simulink model "CopterSim3DEnvironment123"  (R2022a)
settings: Solver=ode4  StartTime=0.0  StopTime=2000  FixedStep=0.001  RelTol=1e-3
PreLoadFcn:
  | filepath  = fileparts(get_param(bdroot, 'FileName'));
  | cd(filepath);
InitFcn:
  | if exist('Init_control.m','file')
  |      Init_control;
  | end
undefined symbols (not defined in the file): d_i, Earth, earthRadius, h_i, KiPitchAttitude, KiPitchRate, KiRollAttitude, KiRollRate, KiYawRate, KpPitchAttitude, KpPitchRate, KpRollAttitude, KpRollRate, KpYawRate, ModelInit_RPM, ModelParam_envAltitude, ModelParam_GlobalNoiseGainSwitch, ModelParam_GPSEphFinal, ModelParam_GPSEpvFinal, ModelParam_GPSEpvInitial, ModelParam_GPSEpvTimeConstant, ModelParam_GPSFix3DFix, ModelParam_GPSSatsVisible, ModelParam_motorCr, ModelParam_motorJm, ModelParam_motorMinThr, ModelParam_motorT, ModelParam_motorWb, ModelParam_noiseBaroCoupleWithSpeed, ModelParam_noiseGPSSampTime, ModelParam_noiseLowPassFilterCoeAccel, ModelParam_noiseLowPassFilterCoeGyro, ModelParam_noisePowerIMU, ModelParam_noisePowerOffGainAccel, ModelParam_noisePowerOffGainAccelZ, ModelParam_noisePowerOffGainGyro, ModelParam_noisePowerOffGainGyroZ, ModelParam_noisePowerOffGainMag, ModelParam_noisePowerOffGainMagZ, ModelParam_noisePowerOnGainAccel, ModelParam_noisePowerOnGainAccelZ, ModelParam_noisePowerOnGainGyro, ModelParam_noisePowerOnGainGyroZ, ModelParam_noisePowerOnGainMag, ModelParam_noisePowerOnGainMagZ, ModelParam_noiseSampleTimeAccel, ModelParam_noiseSampleTimeGyro, ModelParam_noiseSampleTimeMag, ModelParam_noiseUpperGPS, ModelParam_noiseUpperWindBodyRatio, ModelParam_noiseWindSampTime, ModelParam_rotorCm, ModelParam_rotorCt, ModelParam_timeSamp, ModelParam_timeSampBaro, ModelParam_uavCCm, ModelParam_uavCd, ModelParam_uavDearo, ModelParam_uavMass, ModelParam_uavR ... (+6)
libraries: simulink x12, slpidlib x5, aerolibfltsims x4, aerolibtransform2 x3, sharedtransform x3, aerolibasang x3, aerolibatmos2 x2, sharedutil x2, aerolibutil x2, etargetslib x2, shared6dof x1, aerolibconvert2 x1
(part 2 of 3)

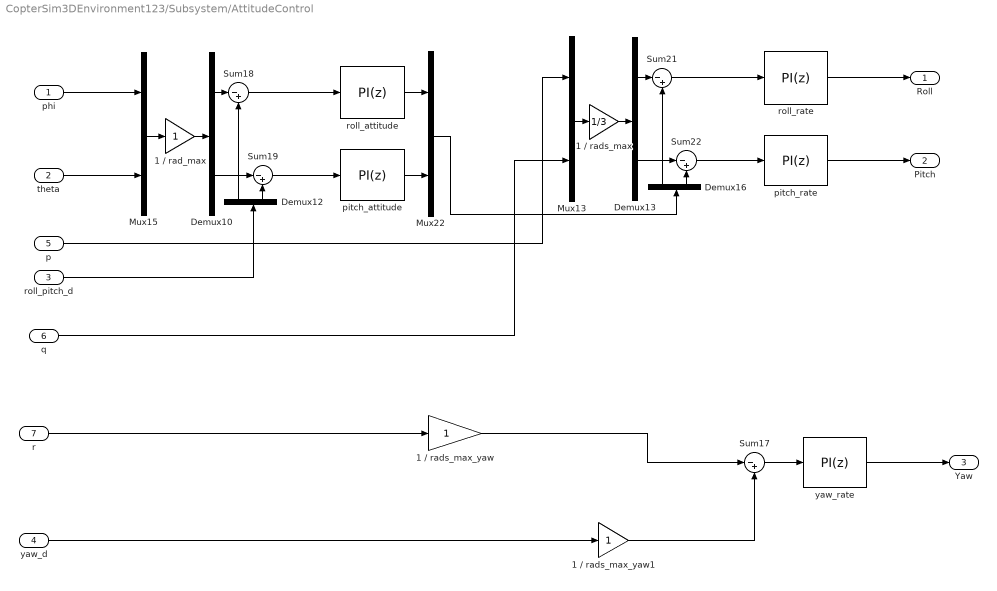
== system CopterSim3DEnvironment123/Subsystem/AttitudeControl ==
  phi : Inport
  theta : Inport  Port=2
  roll_pitch_d : Inport  Port=3
  yaw_d : Inport  Port=4
  p : Inport  Port=5
  q : Inport  Port=6
  r : Inport  Port=7
  1 / rad_max : Gain
  1 / rads_max : Gain  Gain=1/3
  1 / rads_max_yaw : Gain
  1 / rads_max_yaw1 : Gain
  Demux{10,12..13,16} (4 alike) : Demux  Outputs=2
  Mux13 : Mux  Inputs=2
  Mux15 : Mux  Inputs=2
  Mux22 : Mux  Inputs=2
  Sum{17..19,21..22} (5 alike) : Sum  Inputs=|-+
  pitch_attitude : slpidlib/PID Controller  Controller=PI  Form=Parallel  TimeDomain=Discrete-time  UseExternalTs=off  SampleTime=-1  IntegratorMethod=Forward Euler  FilterMethod=Forward Euler  ControllerParametersSource=internal  P=KpPitchAttitude  I=KiPitchAttitude  UseKiTs=off  D=0.01  N=100  UseFilter=on  TunerSelectOption=Transfer Function Based (PID Tuner App)  InitialConditionSource=internal  InitialConditionForIntegrator=0  InitialConditionForFilter=0  DifferentiatorICPrevScaledInput=0  ExternalReset=none  TrackingMode=off  Kt=1  LimitOutput=on  SatLimitsSource=internal  UpperSaturationLimit=1  LowerSaturationLimit=-1  LinearizeAsGain=on  AntiWindupMode=back-calculation  Kb=1  POutMin=[]  POutMax=[]  IOutMin=[]  IOutMax=[]  DOutMin=[]  DOutMax=[]  NOutMin=[]  NOutMax=[]  SumOutMin=[]  SumOutMax=[]  SaturationOutMin=[]  SaturationOutMax=[]  PParamMin=[]  PParamMax=[]  IParamMin=[]  IParamMax=[]  DParamMin=[]  DParamMax=[]  NParamMin=[]  NParamMax=[]  KbParamMin=[]  KbParamMax=[]  KtParamMin=[]  KtParamMax=[]  KbOutMin=[]  KbOutMax=[]  KtOutMin=[]  KtOutMax=[]  IntegratorOutMin=[]  IntegratorOutMax=[]  FilterOutMin=[]  FilterOutMax=[]  SumI1OutMin=[]  SumI1OutMax=[]  SumI2OutMin=[]  SumI2OutMax=[]  SumI3OutMin=[]  SumI3OutMax=[]  SumI4OutMin=[]  SumI4OutMax=[]  SumDOutMin=[]  SumDOutMax=[]  DifferentiatorOutMin=[]  DifferentiatorOutMax=[]  FilterDiffOutCoefMin=[]  FilterDiffOutCoefMax=[]  ReciprocalOutMin=[]  ReciprocalOutMax=[]  SumDenOutMin=[]  SumDenOutMax=[]  SumNumOutMin=[]  SumNumOutMax=[]  DivideOutMin=[]  DivideOutMax=[]  UdiffTsProdOutMin=[]  UdiffTsProdOutMax=[]  NTsProdOutMin=[]  NTsProdOutMax=[]  UintegralTsProdOutMin=[]  UintegralTsProdOutMax=[]  UngainTsProdOutMin=[]  UngainTsProdOutMax=[]  IntegratorContinuousStateAttributes=''  IntegratorStateMustResolveToSignalObject=off  IntegratorRTWStateStorageClass=Auto  FilterContinuousStateAttributes=''  FilterStateMustResolveToSignalObject=off  FilterRTWStateStorageClass=Auto  ParallelPVariant=InternalParameters  IdealPVariant=Disabled  IVariant=InternalParameters  DVariant=Disabled  IntegratorVariant=Discrete  SatVariant=Enabled  AWVariant=BackCalculation  PCopyVariant=Disabled  TRVariant=Disabled  FdbkBlocksVariant=Forward  IdealPFdbkVariant=Disabled  SatFdbkVariant=Disabled  DerivativeFilterVariant=Disabled  NVariant=Disabled  NCopyVariant=Disabled_SignalSpec  FilterICVariant=Disabled  IntegratorICVariant=InternalICs  ExternalResetVariant=Disabled  TRSumVariant=Passthrough  SumFdbkVariant=Disabled  SumVariant=Sum_PI  TsampFilterVariant=InternalTs  TsampNgainVariant=Passthrough  TsampIntegralVariant=Passthrough  ExternalSaturationOutDataTypeStr=Inherit: Same as second input  aMode=0
  pitch_rate : slpidlib/PID Controller  Controller=PI  Form=Parallel  TimeDomain=Discrete-time  UseExternalTs=off  SampleTime=-1  IntegratorMethod=Forward Euler  FilterMethod=Forward Euler  ControllerParametersSource=internal  P=KpPitchRate  I=KiPitchRate  UseKiTs=off  D=0.0024  N=100  UseFilter=on  TunerSelectOption=Transfer Function Based (PID Tuner App)  InitialConditionSource=internal  InitialConditionForIntegrator=0  InitialConditionForFilter=0  DifferentiatorICPrevScaledInput=0  ExternalReset=none  TrackingMode=off  Kt=1  LimitOutput=on  SatLimitsSource=internal  UpperSaturationLimit=1  LowerSaturationLimit=-1  LinearizeAsGain=on  AntiWindupMode=back-calculation  Kb=1  POutMin=[]  POutMax=[]  IOutMin=[]  IOutMax=[]  DOutMin=[]  DOutMax=[]  NOutMin=[]  NOutMax=[]  SumOutMin=[]  SumOutMax=[]  SaturationOutMin=[]  SaturationOutMax=[]  PParamMin=[]  PParamMax=[]  IParamMin=[]  IParamMax=[]  DParamMin=[]  DParamMax=[]  NParamMin=[]  NParamMax=[]  KbParamMin=[]  KbParamMax=[]  KtParamMin=[]  KtParamMax=[]  KbOutMin=[]  KbOutMax=[]  KtOutMin=[]  KtOutMax=[]  IntegratorOutMin=[]  IntegratorOutMax=[]  FilterOutMin=[]  FilterOutMax=[]  SumI1OutMin=[]  SumI1OutMax=[]  SumI2OutMin=[]  SumI2OutMax=[]  SumI3OutMin=[]  SumI3OutMax=[]  SumI4OutMin=[]  SumI4OutMax=[]  SumDOutMin=[]  SumDOutMax=[]  DifferentiatorOutMin=[]  DifferentiatorOutMax=[]  FilterDiffOutCoefMin=[]  FilterDiffOutCoefMax=[]  ReciprocalOutMin=[]  ReciprocalOutMax=[]  SumDenOutMin=[]  SumDenOutMax=[]  SumNumOutMin=[]  SumNumOutMax=[]  DivideOutMin=[]  DivideOutMax=[]  UdiffTsProdOutMin=[]  UdiffTsProdOutMax=[]  NTsProdOutMin=[]  NTsProdOutMax=[]  UintegralTsProdOutMin=[]  UintegralTsProdOutMax=[]  UngainTsProdOutMin=[]  UngainTsProdOutMax=[]  IntegratorContinuousStateAttributes=''  IntegratorStateMustResolveToSignalObject=off  IntegratorRTWStateStorageClass=Auto  FilterContinuousStateAttributes=''  FilterStateMustResolveToSignalObject=off  FilterRTWStateStorageClass=Auto  ParallelPVariant=InternalParameters  IdealPVariant=Disabled  IVariant=InternalParameters  DVariant=Disabled  IntegratorVariant=Discrete  SatVariant=Enabled  AWVariant=BackCalculation  PCopyVariant=Disabled  TRVariant=Disabled  FdbkBlocksVariant=Forward  IdealPFdbkVariant=Disabled  SatFdbkVariant=Disabled  DerivativeFilterVariant=Disabled  NVariant=Disabled  NCopyVariant=Disabled_SignalSpec  FilterICVariant=Disabled  IntegratorICVariant=InternalICs  ExternalResetVariant=Disabled  TRSumVariant=Passthrough  SumFdbkVariant=Disabled  SumVariant=Sum_PI  TsampFilterVariant=InternalTs  TsampNgainVariant=Passthrough  TsampIntegralVariant=Passthrough  ExternalSaturationOutDataTypeStr=Inherit: Same as second input  aMode=0
  roll_attitude : slpidlib/PID Controller  Controller=PI  Form=Parallel  TimeDomain=Discrete-time  UseExternalTs=off  SampleTime=-1  IntegratorMethod=Forward Euler  FilterMethod=Forward Euler  ControllerParametersSource=internal  P=KpRollAttitude  I=KiRollAttitude  UseKiTs=off  D=0.01  N=100  UseFilter=on  TunerSelectOption=Transfer Function Based (PID Tuner App)  InitialConditionSource=internal  InitialConditionForIntegrator=0  InitialConditionForFilter=0  DifferentiatorICPrevScaledInput=0  ExternalReset=none  TrackingMode=off  Kt=1  LimitOutput=on  SatLimitsSource=internal  UpperSaturationLimit=1  LowerSaturationLimit=-1  LinearizeAsGain=on  AntiWindupMode=back-calculation  Kb=1  POutMin=[]  POutMax=[]  IOutMin=[]  IOutMax=[]  DOutMin=[]  DOutMax=[]  NOutMin=[]  NOutMax=[]  SumOutMin=[]  SumOutMax=[]  SaturationOutMin=[]  SaturationOutMax=[]  PParamMin=[]  PParamMax=[]  IParamMin=[]  IParamMax=[]  DParamMin=[]  DParamMax=[]  NParamMin=[]  NParamMax=[]  KbParamMin=[]  KbParamMax=[]  KtParamMin=[]  KtParamMax=[]  KbOutMin=[]  KbOutMax=[]  KtOutMin=[]  KtOutMax=[]  IntegratorOutMin=[]  IntegratorOutMax=[]  FilterOutMin=[]  FilterOutMax=[]  SumI1OutMin=[]  SumI1OutMax=[]  SumI2OutMin=[]  SumI2OutMax=[]  SumI3OutMin=[]  SumI3OutMax=[]  SumI4OutMin=[]  SumI4OutMax=[]  SumDOutMin=[]  SumDOutMax=[]  DifferentiatorOutMin=[]  DifferentiatorOutMax=[]  FilterDiffOutCoefMin=[]  FilterDiffOutCoefMax=[]  ReciprocalOutMin=[]  ReciprocalOutMax=[]  SumDenOutMin=[]  SumDenOutMax=[]  SumNumOutMin=[]  SumNumOutMax=[]  DivideOutMin=[]  DivideOutMax=[]  UdiffTsProdOutMin=[]  UdiffTsProdOutMax=[]  NTsProdOutMin=[]  NTsProdOutMax=[]  UintegralTsProdOutMin=[]  UintegralTsProdOutMax=[]  UngainTsProdOutMin=[]  UngainTsProdOutMax=[]  IntegratorContinuousStateAttributes=''  IntegratorStateMustResolveToSignalObject=off  IntegratorRTWStateStorageClass=Auto  FilterContinuousStateAttributes=''  FilterStateMustResolveToSignalObject=off  FilterRTWStateStorageClass=Auto  ParallelPVariant=InternalParameters  IdealPVariant=Disabled  IVariant=InternalParameters  DVariant=Disabled  IntegratorVariant=Discrete  SatVariant=Enabled  AWVariant=BackCalculation  PCopyVariant=Disabled  TRVariant=Disabled  FdbkBlocksVariant=Forward  IdealPFdbkVariant=Disabled  SatFdbkVariant=Disabled  DerivativeFilterVariant=Disabled  NVariant=Disabled  NCopyVariant=Disabled_SignalSpec  FilterICVariant=Disabled  IntegratorICVariant=InternalICs  ExternalResetVariant=Disabled  TRSumVariant=Passthrough  SumFdbkVariant=Disabled  SumVariant=Sum_PI  TsampFilterVariant=InternalTs  TsampNgainVariant=Passthrough  TsampIntegralVariant=Passthrough  ExternalSaturationOutDataTypeStr=Inherit: Same as second input  aMode=0
  roll_rate : slpidlib/PID Controller  Controller=PI  Form=Parallel  TimeDomain=Discrete-time  UseExternalTs=off  SampleTime=-1  IntegratorMethod=Forward Euler  FilterMethod=Forward Euler  ControllerParametersSource=internal  P=KpRollRate  I=KiRollRate  UseKiTs=off  D=0.0024  N=100  UseFilter=on  TunerSelectOption=Transfer Function Based (PID Tuner App)  InitialConditionSource=internal  InitialConditionForIntegrator=0  InitialConditionForFilter=0  DifferentiatorICPrevScaledInput=0  ExternalReset=none  TrackingMode=off  Kt=1  LimitOutput=on  SatLimitsSource=internal  UpperSaturationLimit=1  LowerSaturationLimit=-1  LinearizeAsGain=on  AntiWindupMode=back-calculation  Kb=1  POutMin=[]  POutMax=[]  IOutMin=[]  IOutMax=[]  DOutMin=[]  DOutMax=[]  NOutMin=[]  NOutMax=[]  SumOutMin=[]  SumOutMax=[]  SaturationOutMin=[]  SaturationOutMax=[]  PParamMin=[]  PParamMax=[]  IParamMin=[]  IParamMax=[]  DParamMin=[]  DParamMax=[]  NParamMin=[]  NParamMax=[]  KbParamMin=[]  KbParamMax=[]  KtParamMin=[]  KtParamMax=[]  KbOutMin=[]  KbOutMax=[]  KtOutMin=[]  KtOutMax=[]  IntegratorOutMin=[]  IntegratorOutMax=[]  FilterOutMin=[]  FilterOutMax=[]  SumI1OutMin=[]  SumI1OutMax=[]  SumI2OutMin=[]  SumI2OutMax=[]  SumI3OutMin=[]  SumI3OutMax=[]  SumI4OutMin=[]  SumI4OutMax=[]  SumDOutMin=[]  SumDOutMax=[]  DifferentiatorOutMin=[]  DifferentiatorOutMax=[]  FilterDiffOutCoefMin=[]  FilterDiffOutCoefMax=[]  ReciprocalOutMin=[]  ReciprocalOutMax=[]  SumDenOutMin=[]  SumDenOutMax=[]  SumNumOutMin=[]  SumNumOutMax=[]  DivideOutMin=[]  DivideOutMax=[]  UdiffTsProdOutMin=[]  UdiffTsProdOutMax=[]  NTsProdOutMin=[]  NTsProdOutMax=[]  UintegralTsProdOutMin=[]  UintegralTsProdOutMax=[]  UngainTsProdOutMin=[]  UngainTsProdOutMax=[]  IntegratorContinuousStateAttributes=''  IntegratorStateMustResolveToSignalObject=off  IntegratorRTWStateStorageClass=Auto  FilterContinuousStateAttributes=''  FilterStateMustResolveToSignalObject=off  FilterRTWStateStorageClass=Auto  ParallelPVariant=InternalParameters  IdealPVariant=Disabled  IVariant=InternalParameters  DVariant=Disabled  IntegratorVariant=Discrete  SatVariant=Enabled  AWVariant=BackCalculation  PCopyVariant=Disabled  TRVariant=Disabled  FdbkBlocksVariant=Forward  IdealPFdbkVariant=Disabled  SatFdbkVariant=Disabled  DerivativeFilterVariant=Disabled  NVariant=Disabled  NCopyVariant=Disabled_SignalSpec  FilterICVariant=Disabled  IntegratorICVariant=InternalICs  ExternalResetVariant=Disabled  TRSumVariant=Passthrough  SumFdbkVariant=Disabled  SumVariant=Sum_PI  TsampFilterVariant=InternalTs  TsampNgainVariant=Passthrough  TsampIntegralVariant=Passthrough  ExternalSaturationOutDataTypeStr=Inherit: Same as second input  aMode=0
  yaw_rate : slpidlib/PID Controller  Controller=PI  Form=Parallel  TimeDomain=Discrete-time  UseExternalTs=off  SampleTime=-1  IntegratorMethod=Forward Euler  FilterMethod=Forward Euler  ControllerParametersSource=internal  P=KpYawRate  I=KiYawRate  UseKiTs=off  D=0  N=100  UseFilter=on  TunerSelectOption=Transfer Function Based (PID Tuner App)  InitialConditionSource=internal  InitialConditionForIntegrator=0  InitialConditionForFilter=0  DifferentiatorICPrevScaledInput=0  ExternalReset=none  TrackingMode=off  Kt=1  LimitOutput=on  SatLimitsSource=internal  UpperSaturationLimit=1  LowerSaturationLimit=-1  LinearizeAsGain=on  AntiWindupMode=back-calculation  Kb=1  POutMin=[]  POutMax=[]  IOutMin=[]  IOutMax=[]  DOutMin=[]  DOutMax=[]  NOutMin=[]  NOutMax=[]  SumOutMin=[]  SumOutMax=[]  SaturationOutMin=[]  SaturationOutMax=[]  PParamMin=[]  PParamMax=[]  IParamMin=[]  IParamMax=[]  DParamMin=[]  DParamMax=[]  NParamMin=[]  NParamMax=[]  KbParamMin=[]  KbParamMax=[]  KtParamMin=[]  KtParamMax=[]  KbOutMin=[]  KbOutMax=[]  KtOutMin=[]  KtOutMax=[]  IntegratorOutMin=[]  IntegratorOutMax=[]  FilterOutMin=[]  FilterOutMax=[]  SumI1OutMin=[]  SumI1OutMax=[]  SumI2OutMin=[]  SumI2OutMax=[]  SumI3OutMin=[]  SumI3OutMax=[]  SumI4OutMin=[]  SumI4OutMax=[]  SumDOutMin=[]  SumDOutMax=[]  DifferentiatorOutMin=[]  DifferentiatorOutMax=[]  FilterDiffOutCoefMin=[]  FilterDiffOutCoefMax=[]  ReciprocalOutMin=[]  ReciprocalOutMax=[]  SumDenOutMin=[]  SumDenOutMax=[]  SumNumOutMin=[]  SumNumOutMax=[]  DivideOutMin=[]  DivideOutMax=[]  UdiffTsProdOutMin=[]  UdiffTsProdOutMax=[]  NTsProdOutMin=[]  NTsProdOutMax=[]  UintegralTsProdOutMin=[]  UintegralTsProdOutMax=[]  UngainTsProdOutMin=[]  UngainTsProdOutMax=[]  IntegratorContinuousStateAttributes=''  IntegratorStateMustResolveToSignalObject=off  IntegratorRTWStateStorageClass=Auto  FilterContinuousStateAttributes=''  FilterStateMustResolveToSignalObject=off  FilterRTWStateStorageClass=Auto  ParallelPVariant=InternalParameters  IdealPVariant=Disabled  IVariant=InternalParameters  DVariant=Disabled  IntegratorVariant=Discrete  SatVariant=Enabled  AWVariant=BackCalculation  PCopyVariant=Disabled  TRVariant=Disabled  FdbkBlocksVariant=Forward  IdealPFdbkVariant=Disabled  SatFdbkVariant=Disabled  DerivativeFilterVariant=Disabled  NVariant=Disabled  NCopyVariant=Disabled_SignalSpec  FilterICVariant=Disabled  IntegratorICVariant=InternalICs  ExternalResetVariant=Disabled  TRSumVariant=Passthrough  SumFdbkVariant=Disabled  SumVariant=Sum_PI  TsampFilterVariant=InternalTs  TsampNgainVariant=Passthrough  TsampIntegralVariant=Passthrough  ExternalSaturationOutDataTypeStr=Inherit: Same as second input  aMode=0
  Roll : Outport  VectorParamsAs1DForOutWhenUnconnected=off
  Pitch : Outport  Port=2  VectorParamsAs1DForOutWhenUnconnected=off
  Yaw : Outport  Port=3  VectorParamsAs1DForOutWhenUnconnected=off
  wires:
  r/1 -> 1 / rads_max_yaw/1
  q/1 -> Mux13/2
  Mux22/1 -> Demux16/1
  yaw_rate/1 -> Yaw/1
  phi/1 -> Mux15/1
  Mux15/1 -> 1 / rad_max/1
  theta/1 -> Mux15/2
  1 / rads_max_yaw/1 -> Sum17/1
  roll_rate/1 -> Roll/1
  Sum19/1 -> pitch_attitude/1
  pitch_attitude/1 -> Mux22/2
  roll_attitude/1 -> Mux22/1
  Demux16/1 -> Sum21/2
  yaw_d/1 -> 1 / rads_max_yaw1/1
  roll_pitch_d/1 -> Demux12/1
  Demux16/2 -> Sum22/2
  Demux12/1 -> Sum18/2
  Demux12/2 -> Sum19/2
  p/1 -> Mux13/1
  Demux10/1 -> Sum18/1
  Demux10/2 -> Sum19/1
  1 / rad_max/1 -> Demux10/1
  Sum18/1 -> roll_attitude/1
  pitch_rate/1 -> Pitch/1
  Mux13/1 -> 1 / rads_max/1
  Sum22/1 -> pitch_rate/1
  Sum17/1 -> yaw_rate/1
  Demux13/1 -> Sum21/1
  Demux13/2 -> Sum22/1
  1 / rads_max/1 -> Demux13/1
  Sum21/1 -> roll_rate/1
  1 / rads_max_yaw1/1 -> Sum17/2

== system CopterSim3DEnvironment123/Subsystem/InputConditioning1 ==
  note: Roll Angle limit: 0.5 rad
  note: Normalization
  roll : Inport
  pitch : Inport  Port=2
  thrust : Inport  Port=3
  yaw : Inport  Port=4
  Fcn2 : Fcn  Expr=(u - 1500)/400
  Fcn5 : Fcn  Expr=(u - 1500)/400
  Fcn6 : Fcn  Expr=(u - 1100) / 800
  Fcn7 : Fcn  Expr=(u - 1500)/400
  Gain1 : Gain  Gain=0.5
  Gain2 : Gain  Gain=[1 1]  OutDataTypeStr=Inherit: Inherit via back propagation
  Gain3 : Gain  Gain=0.5
  Gain4 : Gain  Gain=0.5
  MATLAB Function : MATLAB Function  TreatAsAtomicUnit=on
  MATLAB Function1 : MATLAB Function  TreatAsAtomicUnit=on
  MATLAB Function2 : MATLAB Function  TreatAsAtomicUnit=on
  MATLAB Function3 : MATLAB Function  TreatAsAtomicUnit=on
  Mux21 : Mux  Inputs=2
  Saturation10 : Saturate  UpperLimit=1  LowerLimit=0
  Saturation7 : Saturate  UpperLimit=1  LowerLimit=-1
  Saturation8 : Saturate  UpperLimit=1  LowerLimit=-1
  Saturation9 : Saturate  UpperLimit=1  LowerLimit=-1
  Roll_Pitch : Outport  VectorParamsAs1DForOutWhenUnconnected=off
  Yaw : Outport  Port=2  VectorParamsAs1DForOutWhenUnconnected=off
  Thrust : Outport  Port=3  VectorParamsAs1DForOutWhenUnconnected=off
  wires:
  Saturation10/1 -> Thrust/1
  Gain2/1 -> Roll_Pitch/1
  Mux21/1 -> Gain2/1
  Saturation8/1 -> Mux21/2
  Fcn6/1 -> Saturation10/1
  Fcn2/1 -> Gain1/1
  Fcn5/1 -> Gain3/1
  Saturation9/1 -> Mux21/1
  Fcn7/1 -> Gain4/1
  pitch/1 -> MATLAB Function2/1(u)
  MATLAB Function1/1(y) -> Fcn7/1
  thrust/1 -> MATLAB Function3/1(u)
  roll/1 -> MATLAB Function/1(u)
  MATLAB Function2/1(y) -> Fcn5/1
  MATLAB Function/1(y) -> Fcn2/1
  yaw/1 -> MATLAB Function1/1(u)
  MATLAB Function3/1(y) -> Fcn6/1
  Saturation7/1 -> Yaw/1
  Gain1/1 -> Saturation9/1
  Gain3/1 -> Saturation8/1
  Gain4/1 -> Saturation7/1

== system CopterSim3DEnvironment123/To FlightGear/Subsystem1 ==
  copterID : Inport  PortDimensions=1
  vehicleType : Inport  Port=2  PortDimensions=1
  PosE : Inport  Port=3  PortDimensions=3
  AngEuler : Inport  Port=4  PortDimensions=3
  pwms : Inport  Port=5
  Clock : Clock
  Constant{,3..5} (4 alike) : Constant  Value=[0,0,0]
  Constant1 : Constant  Value=[0,0,0,0]
  Subsystem : Subsystem
  toUnReal : Outport  VectorParamsAs1DForOutWhenUnconnected=off
  wires:
  Constant/1 -> Subsystem/4("VelE ")
  PosE/1 -> Subsystem/5(PosE)
  vehicleType/1 -> Subsystem/2(vehicleType)
  Clock/1 -> Subsystem/3(runnedTime)
  Constant4/1 -> Subsystem/10(RateB)
  Constant5/1 -> Subsystem/11(PosGPS)
  AngEuler/1 -> Subsystem/6(AngEuler)
  Subsystem/1(toUnReal) -> toUnReal/1
  Constant3/1 -> Subsystem/9(AccB)
  Constant1/1 -> Subsystem/7(AngQuatern)
  copterID/1 -> Subsystem/1(copterID)
  pwms/1 -> Subsystem/8(MotorRPMS)

== system CopterSim3DEnvironment123/Quadcopter Dynamics/Force and Moment Model/Propeller Model ==
  uavType : Inport
  MotorRads : Inport  Port=2
  uavR : Inport  Port=3
  uavDearo : Inport  Port=4
  Cm : Inport  Port=5
  Ct : Inport  Port=6
  Jm : Inport  Port=7
  wb : Inport  Port=8
  Vb : Inport  Port=9
  Cd : Inport  Port=10
  Car : Subsystem  TreatAsAtomicUnit=on
  If : If  IfExpression=u1 >= 50
  Multicopter : Subsystem  TreatAsAtomicUnit=on
  Switch : Switch  Threshold=50  SaturateOnIntegerOverflow=off  InputSameDT=off
  Switch1 : Switch  Threshold=50  SaturateOnIntegerOverflow=off  InputSameDT=off
  Terminator : Terminator
  Terminator1 : Terminator
  Fb : Outport  VectorParamsAs1DForOutWhenUnconnected=off
  Mb : Outport  Port=2  VectorParamsAs1DForOutWhenUnconnected=off
  wires:
  Vb/1 -> Terminator/1
  Cd/1 -> Terminator1/1
  uavType/1 -> If/1, Switch/2, Switch1/2, Multicopter/1(uavType)
  Switch/1 -> Fb/1
  Switch1/1 -> Mb/1
  If/2 -> Multicopter/Action
  If/1 -> Car/Action
  Car/1(Fb) -> Switch/1
  Multicopter/1(Fb) -> Switch/3
  Car/2(Mb) -> Switch1/1
  Multicopter/2(Mb) -> Switch1/3
  MotorRads/1 -> Car/1(MotorRads), Multicopter/2(MotorRads)
  uavDearo/1 -> Multicopter/4(uavDearo)
  Cm/1 -> Multicopter/5(Cm)
  Ct/1 -> Multicopter/6(Ct)
  Jm/1 -> Multicopter/7(Jm)
  wb/1 -> Multicopter/8(wb)
  uavR/1 -> Multicopter/3(uavR)

== system CopterSim3DEnvironment123/Quadcopter Dynamics/Motor Model/MotorNonlinearDynamic1 ==
  Wb : Inport
  Cr : Inport  Port=2
  motorT : Inport  Port=3
  ModelInit_RPM : Inport  Port=4
  PWM : Inport  Port=5
  Minimum Throttle Cutoff : simulink/Logic and Bit Operations/Compare To Constant  relop=>=  const=ModelParam_motorMinThr  OutDataTypeStr=uint8
  Motor_Dynamics : Subsystem  TreatAsAtomicUnit=on
  Motor_Dynamics_backup : StateSpace  Commented=on  A=-1/ModelParam_motorT  C=1/ModelParam_motorT  D=0  InitialCondition=ModelInit_RPM*ModelParam_motorT
  Product : Product
  Product1 : Product
  Signal_Saturation : Saturate  UpperLimit=0.95  LowerLimit=0
  Sum1 : Sum  Inputs=++|
  radW : Outport  VectorParamsAs1DForOutWhenUnconnected=off
  wires:
  PWM/1 -> Signal_Saturation/1
  Motor_Dynamics/1(motor_rate_act) -> radW/1
  Product/1 -> Motor_Dynamics/1(motor_rate_d)
  Signal_Saturation/1 -> Product1/2, Minimum Throttle Cutoff/1
  Product1/1 -> Sum1/2
  Sum1/1 -> Product/1
  Wb/1 -> Sum1/1
  Minimum Throttle Cutoff/1 -> Product/2
  Cr/1 -> Product1/1
  motorT/1 -> Motor_Dynamics/3(motorT)
  ModelInit_RPM/1 -> Motor_Dynamics/2(ModelInit_RPM)

== system CopterSim3DEnvironment123/Quadcopter Dynamics/Motor Model/MotorNonlinearDynamic2 ==
  Wb : Inport
  Cr : Inport  Port=2
  motorT : Inport  Port=3
  ModelInit_RPM : Inport  Port=4
  PWM : Inport  Port=5
  Minimum Throttle Cutoff : simulink/Logic and Bit Operations/Compare To Constant  relop=>=  const=ModelParam_motorMinThr  OutDataTypeStr=uint8
  Motor_Dynamics : Subsystem  TreatAsAtomicUnit=on
  Motor_Dynamics_backup : StateSpace  Commented=on  A=-1/ModelParam_motorT  C=1/ModelParam_motorT  D=0  InitialCondition=ModelInit_RPM*ModelParam_motorT
  Product : Product
  Product1 : Product
  Signal_Saturation : Saturate  UpperLimit=0.95  LowerLimit=0
  Sum1 : Sum  Inputs=++|
  radW : Outport  VectorParamsAs1DForOutWhenUnconnected=off
  wires:
  ModelInit_RPM/1 -> Motor_Dynamics/2(ModelInit_RPM)
  motorT/1 -> Motor_Dynamics/3(motorT)
  Cr/1 -> Product1/1
  Minimum Throttle Cutoff/1 -> Product/2
  Wb/1 -> Sum1/1
  Sum1/1 -> Product/1
  Product1/1 -> Sum1/2
  Signal_Saturation/1 -> Minimum Throttle Cutoff/1, Product1/2
  Product/1 -> Motor_Dynamics/1(motor_rate_d)
  Motor_Dynamics/1(motor_rate_act) -> radW/1
  PWM/1 -> Signal_Saturation/1

== system CopterSim3DEnvironment123/Quadcopter Dynamics/Motor Model/MotorNonlinearDynamic3 ==
  Wb : Inport
  Cr : Inport  Port=2
  motorT : Inport  Port=3
  ModelInit_RPM : Inport  Port=4
  PWM : Inport  Port=5
  Minimum Throttle Cutoff : simulink/Logic and Bit Operations/Compare To Constant  relop=>=  const=ModelParam_motorMinThr  OutDataTypeStr=uint8
  Motor_Dynamics : Subsystem  TreatAsAtomicUnit=on
  Motor_Dynamics_backup : StateSpace  Commented=on  A=-1/ModelParam_motorT  C=1/ModelParam_motorT  D=0  InitialCondition=ModelInit_RPM*ModelParam_motorT
  Product : Product
  Product1 : Product
  Signal_Saturation : Saturate  UpperLimit=0.95  LowerLimit=0
  Sum1 : Sum  Inputs=++|
  radW : Outport  VectorParamsAs1DForOutWhenUnconnected=off
  wires:
  PWM/1 -> Signal_Saturation/1
  Motor_Dynamics/1(motor_rate_act) -> radW/1
  Product/1 -> Motor_Dynamics/1(motor_rate_d)
  Signal_Saturation/1 -> Product1/2, Minimum Throttle Cutoff/1
  Product1/1 -> Sum1/2
  Sum1/1 -> Product/1
  Wb/1 -> Sum1/1
  Minimum Throttle Cutoff/1 -> Product/2
  Cr/1 -> Product1/1
  motorT/1 -> Motor_Dynamics/3(motorT)
  ModelInit_RPM/1 -> Motor_Dynamics/2(ModelInit_RPM)

== system CopterSim3DEnvironment123/Quadcopter Dynamics/Motor Model/MotorNonlinearDynamic4 ==
  Wb : Inport
  Cr : Inport  Port=2
  motorT : Inport  Port=3
  ModelInit_RPM : Inport  Port=4
  PWM : Inport  Port=5
  Minimum Throttle Cutoff : simulink/Logic and Bit Operations/Compare To Constant  relop=>=  const=ModelParam_motorMinThr  OutDataTypeStr=uint8
  Motor_Dynamics : Subsystem  TreatAsAtomicUnit=on
  Motor_Dynamics_backup : StateSpace  Commented=on  A=-1/ModelParam_motorT  C=1/ModelParam_motorT  D=0  InitialCondition=ModelInit_RPM*ModelParam_motorT
  Product : Product
  Product1 : Product
  Signal_Saturation : Saturate  UpperLimit=0.95  LowerLimit=0
  Sum1 : Sum  Inputs=++|
  radW : Outport  VectorParamsAs1DForOutWhenUnconnected=off
  wires:
  ModelInit_RPM/1 -> Motor_Dynamics/2(ModelInit_RPM)
  motorT/1 -> Motor_Dynamics/3(motorT)
  Cr/1 -> Product1/1
  Minimum Throttle Cutoff/1 -> Product/2
  Wb/1 -> Sum1/1
  Sum1/1 -> Product/1
  Product1/1 -> Sum1/2
  Signal_Saturation/1 -> Minimum Throttle Cutoff/1, Product1/2
  Product/1 -> Motor_Dynamics/1(motor_rate_d)
  Motor_Dynamics/1(motor_rate_act) -> radW/1
  PWM/1 -> Signal_Saturation/1

== system CopterSim3DEnvironment123/Quadcopter Dynamics/Motor Model/MotorNonlinearDynamic5 ==
  Wb : Inport
  Cr : Inport  Port=2
  motorT : Inport  Port=3
  ModelInit_RPM : Inport  Port=4
  PWM : Inport  Port=5
  Minimum Throttle Cutoff : simulink/Logic and Bit Operations/Compare To Constant  relop=>=  const=ModelParam_motorMinThr  OutDataTypeStr=uint8
  Motor_Dynamics : Subsystem  TreatAsAtomicUnit=on
  Motor_Dynamics_backup : StateSpace  Commented=on  A=-1/ModelParam_motorT  C=1/ModelParam_motorT  D=0  InitialCondition=ModelInit_RPM*ModelParam_motorT
  Product : Product
  Product1 : Product
  Signal_Saturation : Saturate  UpperLimit=0.95  LowerLimit=0
  Sum1 : Sum  Inputs=++|
  radW : Outport  VectorParamsAs1DForOutWhenUnconnected=off
  wires:
  PWM/1 -> Signal_Saturation/1
  Motor_Dynamics/1(motor_rate_act) -> radW/1
  Product/1 -> Motor_Dynamics/1(motor_rate_d)
  Signal_Saturation/1 -> Product1/2, Minimum Throttle Cutoff/1
  Product1/1 -> Sum1/2
  Sum1/1 -> Product/1
  Wb/1 -> Sum1/1
  Minimum Throttle Cutoff/1 -> Product/2
  Cr/1 -> Product1/1
  motorT/1 -> Motor_Dynamics/3(motorT)
  ModelInit_RPM/1 -> Motor_Dynamics/2(ModelInit_RPM)

== system CopterSim3DEnvironment123/Quadcopter Dynamics/Motor Model/MotorNonlinearDynamic6 ==
  Wb : Inport
  Cr : Inport  Port=2
  motorT : Inport  Port=3
  ModelInit_RPM : Inport  Port=4
  PWM : Inport  Port=5
  Minimum Throttle Cutoff : simulink/Logic and Bit Operations/Compare To Constant  relop=>=  const=ModelParam_motorMinThr  OutDataTypeStr=uint8
  Motor_Dynamics : Subsystem  TreatAsAtomicUnit=on
  Motor_Dynamics_backup : StateSpace  Commented=on  A=-1/ModelParam_motorT  C=1/ModelParam_motorT  D=0  InitialCondition=ModelInit_RPM*ModelParam_motorT
  Product : Product
  Product1 : Product
  Signal_Saturation : Saturate  UpperLimit=0.95  LowerLimit=0
  Sum1 : Sum  Inputs=++|
  radW : Outport  VectorParamsAs1DForOutWhenUnconnected=off
  wires:
  ModelInit_RPM/1 -> Motor_Dynamics/2(ModelInit_RPM)
  motorT/1 -> Motor_Dynamics/3(motorT)
  Cr/1 -> Product1/1
  Minimum Throttle Cutoff/1 -> Product/2
  Wb/1 -> Sum1/1
  Sum1/1 -> Product/1
  Product1/1 -> Sum1/2
  Signal_Saturation/1 -> Minimum Throttle Cutoff/1, Product1/2
  Product/1 -> Motor_Dynamics/1(motor_rate_d)
  Motor_Dynamics/1(motor_rate_act) -> radW/1
  PWM/1 -> Signal_Saturation/1

== system CopterSim3DEnvironment123/Quadcopter Dynamics/Motor Model/MotorNonlinearDynamic7 ==
  Wb : Inport
  Cr : Inport  Port=2
  motorT : Inport  Port=3
  ModelInit_RPM : Inport  Port=4
  PWM : Inport  Port=5
  Minimum Throttle Cutoff : simulink/Logic and Bit Operations/Compare To Constant  relop=>=  const=ModelParam_motorMinThr  OutDataTypeStr=uint8
  Motor_Dynamics : Subsystem  TreatAsAtomicUnit=on
  Motor_Dynamics_backup : StateSpace  Commented=on  A=-1/ModelParam_motorT  C=1/ModelParam_motorT  D=0  InitialCondition=ModelInit_RPM*ModelParam_motorT
  Product : Product
  Product1 : Product
  Signal_Saturation : Saturate  UpperLimit=0.95  LowerLimit=0
  Sum1 : Sum  Inputs=++|
  radW : Outport  VectorParamsAs1DForOutWhenUnconnected=off
  wires:
  PWM/1 -> Signal_Saturation/1
  Motor_Dynamics/1(motor_rate_act) -> radW/1
  Product/1 -> Motor_Dynamics/1(motor_rate_d)
  Signal_Saturation/1 -> Product1/2, Minimum Throttle Cutoff/1
  Product1/1 -> Sum1/2
  Sum1/1 -> Product/1
  Wb/1 -> Sum1/1
  Minimum Throttle Cutoff/1 -> Product/2
  Cr/1 -> Product1/1
  motorT/1 -> Motor_Dynamics/3(motorT)
  ModelInit_RPM/1 -> Motor_Dynamics/2(ModelInit_RPM)

== system CopterSim3DEnvironment123/Quadcopter Dynamics/Motor Model/MotorNonlinearDynamic8 ==
  Wb : Inport
  Cr : Inport  Port=2
  motorT : Inport  Port=3
  ModelInit_RPM : Inport  Port=4
  PWM : Inport  Port=5
  Minimum Throttle Cutoff : simulink/Logic and Bit Operations/Compare To Constant  relop=>=  const=ModelParam_motorMinThr  OutDataTypeStr=uint8
  Motor_Dynamics : Subsystem  TreatAsAtomicUnit=on
  Motor_Dynamics_backup : StateSpace  Commented=on  A=-1/ModelParam_motorT  C=1/ModelParam_motorT  D=0  InitialCondition=ModelInit_RPM*ModelParam_motorT
  Product : Product
  Product1 : Product
  Signal_Saturation : Saturate  UpperLimit=0.95  LowerLimit=0
  Sum1 : Sum  Inputs=++|
  radW : Outport  VectorParamsAs1DForOutWhenUnconnected=off
  wires:
  ModelInit_RPM/1 -> Motor_Dynamics/2(ModelInit_RPM)
  motorT/1 -> Motor_Dynamics/3(motorT)
  Cr/1 -> Product1/1
  Minimum Throttle Cutoff/1 -> Product/2
  Wb/1 -> Sum1/1
  Sum1/1 -> Product/1
  Product1/1 -> Sum1/2
  Signal_Saturation/1 -> Minimum Throttle Cutoff/1, Product1/2
  Product/1 -> Motor_Dynamics/1(motor_rate_d)
  Motor_Dynamics/1(motor_rate_act) -> radW/1
  PWM/1 -> Signal_Saturation/1

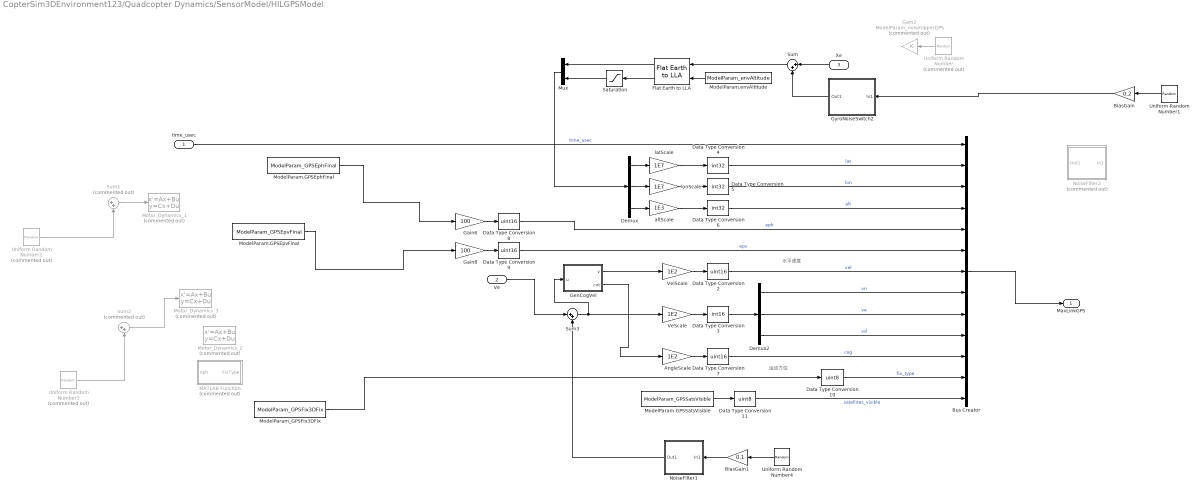
== system CopterSim3DEnvironment123/Quadcopter Dynamics/SensorModel/HILGPSModel ==
  note: 水平速度
  note: 运动方位
  time_usec : Inport
  Ve : Inport  Port=2
  Xe : Inport  Port=3
  AngleScale : Gain  Gain=1E2
  BiasGain : Gain  Gain=0.2
  BiasGain1 : Gain  Gain=0.1
  Bus Creator : BusCreator  Inputs=13  OutDataTypeStr=Bus: MavLinkGPS  NonVirtualBus=on
  Data Type Conversion10 : DataTypeConversion  OutDataTypeStr=uint8  RndMeth=Round  SaturateOnIntegerOverflow=off
  Data Type Conversion11 : DataTypeConversion  OutDataTypeStr=uint8  RndMeth=Round  SaturateOnIntegerOverflow=off
  Data Type Conversion{2,7..9} (4 alike) : DataTypeConversion  OutDataTypeStr=uint16  RndMeth=Round  SaturateOnIntegerOverflow=off
  Data Type Conversion3 : DataTypeConversion  OutDataTypeStr=int16  RndMeth=Round  SaturateOnIntegerOverflow=off
  Data Type Conversion4 : DataTypeConversion  OutDataTypeStr=int32  RndMeth=Round  SaturateOnIntegerOverflow=off
  Data Type Conversion5 : DataTypeConversion  OutDataTypeStr=int32  RndMeth=Round  SaturateOnIntegerOverflow=off
  Data Type Conversion6 : DataTypeConversion  OutDataTypeStr=int32  RndMeth=Round  SaturateOnIntegerOverflow=off
  Demux : Demux  Outputs=3
  Demux2 : Demux  Outputs=3
  Flat Earth to LLA : aerolibtransform2/Flat Earth to LLA  units=Metric (MKS)  ptype=Earth (WGS84)  F=1/298.257223563  R=6378137  refPosPort=off  LL0=ModelParam_GPSLatLong  psi=0
  Gain2 : Gain  Commented=on  Gain=ModelParam_noiseUpperGPS
  Gain6 : Gain  Gain=100
  Gain8 : Gain  Gain=100
  GenCogVel : MATLAB Function  TreatAsAtomicUnit=on
  GyroNoiseSwitch2 : Subsystem
  MATLAB Function : MATLAB Function  Commented=on  TreatAsAtomicUnit=on
  ModelParam.GPSEphFinal : Constant  Value=ModelParam_GPSEphFinal
  ModelParam.GPSEpvFinal : Constant  Value=ModelParam_GPSEpvFinal
  ModelParam.GPSSatsVisible : Constant  Value=ModelParam_GPSSatsVisible
  ModelParam.envAltitude : Constant  Value=ModelParam_envAltitude
  ModelParam_GPSFix3DFix : Constant  Value=ModelParam_GPSFix3DFix
  Motor_Dynamics_1 : StateSpace  Commented=on  A=-1/0.2  C=1/0.2  D=0  InitialCondition=20*0.2
  Motor_Dynamics_2 : StateSpace  Commented=on  A=-1/ModelParam_GPSEpvTimeConstant  C=1/ModelParam_GPSEpvTimeConstant  D=0  InitialCondition=ModelParam_GPSEpvInitial*ModelParam_GPSEpvTimeConstant
  Motor_Dynamics_3 : StateSpace  Commented=on  A=-1/0.2  C=1/0.2  D=0  InitialCondition=20*0.2
  Mux : Mux  Inputs=2
  NoiseFilter1 : Subsystem
  NoiseFilter2 : Subsystem  Commented=on
  Saturation : Saturate  UpperLimit=100000  LowerLimit=0
  Sum : Sum  Inputs=|++
  Sum1 : Sum  Commented=on  Inputs=|++
  Sum2 : Sum  Commented=on  Inputs=|++
  Sum3 : Sum  Inputs=|++
  Uniform Random Number : UniformRandomNumber  Commented=on  Minimum=[-1,-1,-3]  Maximum=[1,1,3]  Seed=[14524,7875,698]  SampleTime=ModelParam_timeSamp
  Uniform Random Number1 : UniformRandomNumber  Minimum=[-1,-1,-2]  Maximum=[1,1,2]  Seed=[1452,787,69]  SampleTime=ModelParam_noiseGPSSampTime
  Uniform Random Number2 : UniformRandomNumber  Commented=on  Minimum=-0.01  Maximum=0.01  Seed=4345454  SampleTime=ModelParam_noiseGPSSampTime
  Uniform Random Number3 : UniformRandomNumber  Commented=on  Seed=3244333  SampleTime=ModelParam_noiseGPSSampTime
  Uniform Random Number4 : UniformRandomNumber  Minimum=[-1,-1,-2]  Maximum=[1,1,2]  Seed=[5445,45433,33433]  SampleTime=ModelParam_noiseGPSSampTime
  VeScale : Gain  Gain=1E2
  VelScale : Gain  Gain=1E2
  altScale : Gain  Gain=1E3
  latScale : Gain  Gain=1E7
  lonScale : Gain  Gain=1E7
  MavLinkGPS : Outport  VectorParamsAs1DForOutWhenUnconnected=off
  wires:
  Data Type Conversion8/1 -> Bus Creator/5  "eph"
  Gain8/1 -> Data Type Conversion9/1
  Gain6/1 -> Data Type Conversion8/1
  Data Type Conversion9/1 -> Bus Creator/6  "epv"
  time_usec/1 -> Bus Creator/1  "time_usec"
  latScale/1 -> Data Type Conversion4/1
  lonScale/1 -> Data Type Conversion5/1
  altScale/1 -> Data Type Conversion6/1
  Data Type Conversion4/1 -> Bus Creator/2  "lat"
  Data Type Conversion5/1 -> Bus Creator/3  "lon"
  Data Type Conversion6/1 -> Bus Creator/4  "alt"
  Demux2/1 -> Bus Creator/8  "vn"
  Demux2/2 -> Bus Creator/9  "ve"
  Demux2/3 -> Bus Creator/10  "vd"
  VeScale/1 -> Data Type Conversion3/1
  Data Type Conversion3/1 -> Demux2/1
  VelScale/1 -> Data Type Conversion2/1
  Data Type Conversion2/1 -> Bus Creator/7  "vel"
  AngleScale/1 -> Data Type Conversion7/1
  Data Type Conversion7/1 -> Bus Creator/11  "cog"
  Data Type Conversion11/1 -> Bus Creator/13  "satellites_visible"
  Data Type Conversion10/1 -> Bus Creator/12  "fix_type"
  ModelParam.GPSSatsVisible/1 -> Data Type Conversion11/1
  Flat Earth to LLA/2 -> Saturation/1
  Saturation/1 -> Mux/2
  ModelParam.envAltitude/1 -> Flat Earth to LLA/2
  Xe/1 -> Sum/1
  Flat Earth to LLA/1 -> Mux/1
  Demux/1 -> latScale/1
  Demux/2 -> lonScale/1
  Demux/3 -> altScale/1
  Uniform Random Number/1 -> Gain2/1
  Sum/1 -> Flat Earth to LLA/1
  Uniform Random Number1/1 -> BiasGain/1
  BiasGain/1 -> GyroNoiseSwitch2/1(In1)
  Mux/1 -> Demux/1
  ModelParam.GPSEphFinal/1 -> Gain6/1
  Sum2/1 -> Motor_Dynamics_3/1
  ModelParam_GPSFix3DFix/1 -> Data Type Conversion10/1
  Ve/1 -> Sum3/1
  GenCogVel/1(v) -> VelScale/1
  GyroNoiseSwitch2/1(Out1) -> Sum/2
  Bus Creator/1 -> MavLinkGPS/1
  BiasGain1/1 -> NoiseFilter1/1(In1)
  Uniform Random Number4/1 -> BiasGain1/1
  GenCogVel/2(cot) -> AngleScale/1
  Sum1/1 -> Motor_Dynamics_1/1
  Uniform Random Number2/1 -> Sum1/2
  Uniform Random Number3/1 -> Sum2/2
  ModelParam.GPSEpvFinal/1 -> Gain8/1
  Sum3/1 -> GenCogVel/1(u), VeScale/1
  NoiseFilter1/1(Out1) -> Sum3/2

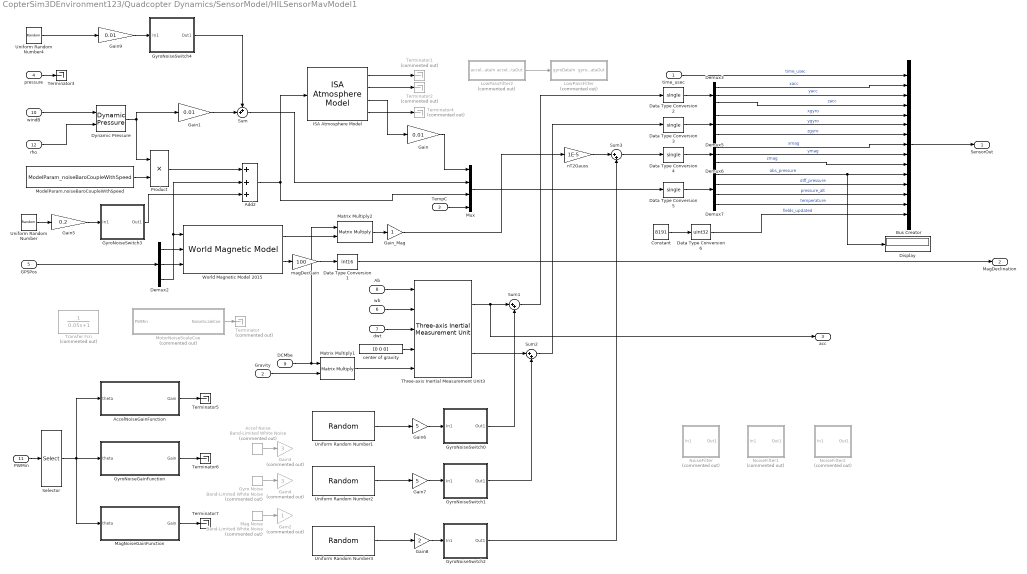
== system CopterSim3DEnvironment123/Quadcopter Dynamics/SensorModel/HILSensorMavModel1 ==
  time_usec : Inport
  Gravity : Inport  Port=2
  TempC : Inport  Port=3
  pressure : Inport  Port=4
  GPSPos : Inport  Port=5
  wb : Inport  Port=6
  dwt : Inport  Port=7
  Ab : Inport  Port=8
  DCMbe : Inport  Port=9
  windB : Inport  Port=10
  PWMin : Inport  Port=11
  rho : Inport  Port=12
  Accel Noise : simulink/Sources/Band-Limited White Noise  Commented=on  Cov=ModelParam_noisePowerAccel  Ts=ModelParam_noiseSampleTimeAccel  seed=[411144,1416,71144]
  AccelNoiseGainFunction : MATLAB Function  TreatAsAtomicUnit=on
  Add2 : Sum  Inputs=+++
  Bus Creator : BusCreator  Inputs=15  OutDataTypeStr=Bus: MavLinkSensor  NonVirtualBus=on
  Constant : Constant  Value=8191
  Data Type Conversion1 : DataTypeConversion  OutDataTypeStr=int16  SaturateOnIntegerOverflow=off  RndMeth=Floor
  Data Type Conversion{2..5} (4 alike) : DataTypeConversion  OutDataTypeStr=single  SaturateOnIntegerOverflow=off  RndMeth=Floor
  Data Type Conversion6 : DataTypeConversion  OutDataTypeStr=uint32  SaturateOnIntegerOverflow=off  RndMeth=Floor
  Demux{2..3,5..6} (4 alike) : Demux  Outputs=3
  Demux7 : Demux
  Display : Display
  Dynamic Pressure : aerolibasang/Dynamic Pressure
  Gain : Gain  Gain=0.01
  Gain1 : Gain  Gain=0.01
  Gain2 : Gain  Commented=on
  Gain3 : Gain  Commented=on  Gain=3
  Gain4 : Gain  Commented=on  Gain=3
  Gain5 : Gain  Gain=0.2
  Gain6 : Gain  Gain=5
  Gain7 : Gain  Gain=5
  Gain8 : Gain  Gain=2
  Gain9 : Gain  Gain=0.01
  Gain_Mag : Gain
  Gyro Noise : simulink/Sources/Band-Limited White Noise  Commented=on  Cov=ModelParam_noisePowerGyro  Ts=ModelParam_noiseSampleTimeGyro  seed=[111,116,144]
  GyroNoiseGainFunction : MATLAB Function  TreatAsAtomicUnit=on
  GyroNoiseSwitch0 : Subsystem
  GyroNoiseSwitch1 : Subsystem
  GyroNoiseSwitch2 : Subsystem
  GyroNoiseSwitch3 : Subsystem
  GyroNoiseSwitch4 : Subsystem
  ISA Atmosphere Model : aerolibatmos2/ISA Atmosphere Model  custom=off  g=9.80665  gamma=1.4  R=287.0531  L=0.0065  h_trop=11000  h_strat=20000  rho0=1.225  P0=101325  T0=288.15  h0=0
  LowPassFilter : Subsystem  Commented=on
  LowPassFilter2 : Subsystem  Commented=on
  Mag Noise : simulink/Sources/Band-Limited White Noise  Commented=on  Cov=ModelParam_noisePowerMag  Ts=ModelParam_noiseSampleTimeMag  seed=[114,11699,999144]
  MagNoiseGainFunction : MATLAB Function  TreatAsAtomicUnit=on
  Matrix Multiply1 : Product  Multiplication=Matrix(*)
  Matrix Multiply2 : Product  Multiplication=Matrix(*)
  ModelParam.noiseBaroCoupleWithSpeed : Constant  Value=ModelParam_noiseBaroCoupleWithSpeed
  MotorNoiseScaleCoe : MATLAB Function  Commented=on  TreatAsAtomicUnit=on
  Mux : Mux
  NoiseFilter : Subsystem  Commented=on
  NoiseFilter1 : Subsystem  Commented=on
  NoiseFilter2 : Subsystem  Commented=on
  Product : Product
  Selector : Selector  InputPortWidth=8  IndexOptions=Index vector (dialog)  Indices=[1]  OutputSizes=1
  Sum : Sum  Inputs=++|
  Sum1 : Sum  Inputs=|++
  Sum2 : Sum  Inputs=|++
  Sum3 : Sum  Inputs=|++
  Terminator{,1..2,4} (4 alike) : Terminator  Commented=on
  Terminator{3,5..7} (4 alike) : Terminator
  Three-axis Inertial Measurement Unit3 : aerolibnav/Three-axis Inertial Measurement Unit  units=Metric (MKS)  imu=[0 0 0]  i_Ts=0  dtype_a=on  w_a=190  z_a=0.707  a_sf_cc=[1 0 0; 0 1 0; 0 0 1]  a_bias=[0 0 0]  a_sat="[-160  -160  -160 160 160 160]"  dtype_g=on  w_g=190  z_g=0.707  g_sf_cc=[1 0 0; 0 1 0; 0 0 1]  g_bias=[0 0 0]  g_sens=[0 0 0]  g_sat="[-4.36  -4.36  -4.36 4.36 4.36 4.36]"  i_rand=off  i_seeds=[23093 23094 23095 23096 23097 23098]  i_pow=ModelParam_noisePowerIMU*[0.0000005 0.0000005 0.0000005 0.000000002 0.000000002 0.000000002]
  Transfer Fcn : TransferFcn  Commented=on  Denominator=[0.05 1]
  Uniform Random Number : UniformRandomNumber  Minimum=-2  Maximum=2  Seed=15634  SampleTime=ModelParam_timeSampBaro
  Uniform Random Number1 : UniformRandomNumber  Minimum=-[0.1,0.1,0.2]  Maximum=[0.1,0.1,0.2]  Seed=[12233,645554,678766]  SampleTime=0.004
  Uniform Random Number2 : UniformRandomNumber  Minimum=-[0.01,0.01,0.01]  Maximum=[0.01,0.01,0.01]  Seed=[3243,44556,2334343]  SampleTime=0.004
  Uniform Random Number3 : UniformRandomNumber  Minimum=-[0.01,0.01,0.01]  Maximum=[0.01,0.01,0.01]  Seed=[45465,454534,1234232]  SampleTime=0.004
  Uniform Random Number4 : UniformRandomNumber  Seed=25634  SampleTime=0.01
  World Magnetic Model 2015 : aerolibgravity2/World Magnetic Model  model=WMM2015 V2 (2015-2020)  customFile='WMM2020.COF'  units=Metric (MKS)  time_in=off  month=November  day=3  year=2017  action=Error  h_out=off  dec_out=on  inc_out=off  ti_out=off
      settings: SourceProductBaseCode=AE
  center of gravity : Constant  Value=[0 0 0]
  magDecGain : Gain  Gain=100
  nT2Gauss : Gain  Gain=1E-5
  SensorOut : Outport  VectorParamsAs1DForOutWhenUnconnected=off
  MagDeclination : Outport  Port=2  VectorParamsAs1DForOutWhenUnconnected=off
  acc : Outport  Port=3  VectorParamsAs1DForOutWhenUnconnected=off
  wires:
  center of gravity/1 -> Three-axis Inertial Measurement Unit3/4
  Sum1/1 -> Data Type Conversion2/1
  Sum2/1 -> Data Type Conversion3/1
  Sum3/1 -> Data Type Conversion4/1
  Matrix Multiply2/1 -> Gain_Mag/1
  magDecGain/1 -> Data Type Conversion1/1
  World Magnetic Model 2015/2 -> magDecGain/1
  GyroNoiseSwitch3/1(Out1) -> Add2/3
  Product/1 -> Add2/1
  ModelParam.noiseBaroCoupleWithSpeed/1 -> Product/2
  rho/1 -> Dynamic Pressure/2
  windB/1 -> Dynamic Pressure/1
  Uniform Random Number/1 -> Gain5/1
  dwt/1 -> Three-axis Inertial Measurement Unit3/3
  Gain_Mag/1 -> nT2Gauss/1
  Dynamic Pressure/1 -> Gain1/1, Product/1
  pressure/1 -> Terminator3/1
  Add2/1 -> Mux/3, ISA Atmosphere Model/1
  Demux2/3 -> World Magnetic Model 2015/1, Add2/2
  Demux2/2 -> World Magnetic Model 2015/3
  Demux2/1 -> World Magnetic Model 2015/2
  Matrix Multiply1/1 -> Three-axis Inertial Measurement Unit3/5
  DCMbe/1 -> Matrix Multiply2/1, Matrix Multiply1/1
  Gravity/1 -> Matrix Multiply1/2
  Sum/1 -> Mux/2
  Gain/1 -> Mux/1
  Data Type Conversion6/1 -> Bus Creator/15  "fields_updated"
  Constant/1 -> Data Type Conversion6/1
  time_usec/1 -> Bus Creator/1  "time_usec"
  GPSPos/1 -> Demux2/1
  Demux7/2 -> Bus Creator/12  "diff_pressure"
  Demux7/3 -> Bus Creator/13  "pressure_alt"
  Demux6/2 -> Bus Creator/9  "ymag"
  Demux6/3 -> Bus Creator/10  "zmag"
  TempC/1 -> Mux/4
  Mux/1 -> Data Type Conversion5/1
  Demux7/1 -> Bus Creator/11, Display/1  "abs_pressure"
  Demux5/2 -> Bus Creator/6  "ygyro"
  Demux6/1 -> Bus Creator/8  "xmag"
  Demux5/3 -> Bus Creator/7  "zgyro"
  Demux7/4 -> Bus Creator/14  "temperature"
  World Magnetic Model 2015/1 -> Matrix Multiply2/2
  Demux3/1 -> Bus Creator/2  "xacc"
  Demux3/2 -> Bus Creator/3  "yacc"
  Demux5/1 -> Bus Creator/5  "xgyro"
  Demux3/3 -> Bus Creator/4  "zacc"
  PWMin/1 -> Selector/1
  Ab/1 -> Three-axis Inertial Measurement Unit3/1
  wb/1 -> Three-axis Inertial Measurement Unit3/2
  MotorNoiseScaleCoe/1(NoiseScaleCoe) -> Terminator/1
  Selector/1 -> AccelNoiseGainFunction/1(theta), MagNoiseGainFunction/1(theta), GyroNoiseGainFunction/1(theta)
  AccelNoiseGainFunction/1(Gain) -> Terminator5/1
  Mag Noise/1 -> Gain2/1
  nT2Gauss/1 -> Sum3/1
  Gain8/1 -> GyroNoiseSwitch2/1(In1)
  GyroNoiseSwitch1/1(Out1) -> Sum2/2
  GyroNoiseSwitch2/1(Out1) -> Sum3/2
  Data Type Conversion2/1 -> Demux3/1
  Data Type Conversion3/1 -> Demux5/1
  Data Type Conversion4/1 -> Demux6/1
  Data Type Conversion5/1 -> Demux7/1
  Bus Creator/1 -> SensorOut/1
  Data Type Conversion1/1 -> MagDeclination/1
  Three-axis Inertial Measurement Unit3/1 -> acc/1, Sum1/1
  Three-axis Inertial Measurement Unit3/2 -> Sum2/1
  ISA Atmosphere Model/2 -> Terminator2/1
  ISA Atmosphere Model/4 -> Terminator4/1
  ISA Atmosphere Model/1 -> Terminator1/1
  Gain5/1 -> GyroNoiseSwitch3/1(In1)
  Accel Noise/1 -> Gain3/1
  GyroNoiseSwitch0/1(Out1) -> Sum1/2
  Gyro Noise/1 -> Gain4/1
  GyroNoiseGainFunction/1(Gain) -> Terminator6/1
  MagNoiseGainFunction/1(Gain) -> Terminator7/1
  Uniform Random Number1/1 -> Gain6/1
  Gain7/1 -> GyroNoiseSwitch1/1(In1)
  Uniform Random Number2/1 -> Gain7/1
  Uniform Random Number3/1 -> Gain8/1
  ISA Atmosphere Model/3 -> Gain/1
  Gain6/1 -> GyroNoiseSwitch0/1(In1)
  LowPassFilter2/1(accelDataOut) -> LowPassFilter/1(gyroDataIn)
  Gain9/1 -> GyroNoiseSwitch4/1(In1)
  Uniform Random Number4/1 -> Gain9/1
  Gain1/1 -> Sum/2
  GyroNoiseSwitch4/1(Out1) -> Sum/1

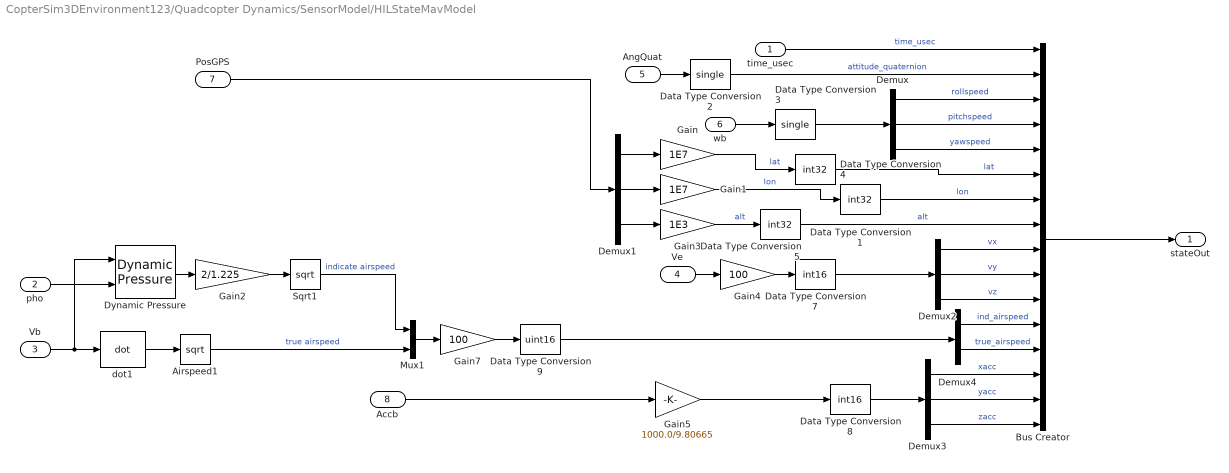
== system CopterSim3DEnvironment123/Quadcopter Dynamics/SensorModel/HILStateMavModel ==
  time_usec : Inport
  pho : Inport  Port=2
  Vb : Inport  Port=3
  Ve : Inport  Port=4
  AngQuat : Inport  Port=5
  wb : Inport  Port=6
  PosGPS : Inport  Port=7
  Accb : Inport  Port=8
  Airspeed1 : Sqrt  AlgorithmType=Newton-Raphson
  Bus Creator : BusCreator  Inputs=16  OutDataTypeStr=Bus: MavLinkStateQuat  NonVirtualBus=on
  Data Type Conversion1 : DataTypeConversion  OutDataTypeStr=int32  RndMeth=Round  SaturateOnIntegerOverflow=off
  Data Type Conversion2 : DataTypeConversion  OutDataTypeStr=single  SaturateOnIntegerOverflow=off  RndMeth=Floor
  Data Type Conversion3 : DataTypeConversion  OutDataTypeStr=single  SaturateOnIntegerOverflow=off  RndMeth=Floor
  Data Type Conversion4 : DataTypeConversion  OutDataTypeStr=int32  RndMeth=Round  SaturateOnIntegerOverflow=off
  Data Type Conversion5 : DataTypeConversion  OutDataTypeStr=int32  RndMeth=Round  SaturateOnIntegerOverflow=off
  Data Type Conversion7 : DataTypeConversion  OutDataTypeStr=int16  RndMeth=Round  SaturateOnIntegerOverflow=off
  Data Type Conversion8 : DataTypeConversion  OutDataTypeStr=int16  RndMeth=Round  SaturateOnIntegerOverflow=off
  Data Type Conversion9 : DataTypeConversion  OutDataTypeStr=uint16  RndMeth=Round  SaturateOnIntegerOverflow=off
  Demux{,1..3} (4 alike) : Demux  Outputs=3
  Demux4 : Demux  Outputs=2
  Dynamic Pressure : aerolibasang/Dynamic Pressure
  Gain : Gain  Gain=1E7
  Gain1 : Gain  Gain=1E7
  Gain2 : Gain  Gain=2/1.225
  Gain3 : Gain  Gain=1E3
  Gain4 : Gain  Gain=100
  Gain5 : Gain  Gain=1000.0/9.80665
  Gain7 : Gain  Gain=100
  Mux1 : Mux  Inputs=2
  Sqrt1 : Sqrt
  dot1 : aerolibasang/Incidence, Sideslip, & Airspeed/dot  SystemSampleTime=-1  VariantActivationTime=update diagram  Latency=0  AutoFrameSizeCalculation=off
      settings: SourceProductBaseCode=AE
  stateOut : Outport  VectorParamsAs1DForOutWhenUnconnected=off
  wires:
  Sqrt1/1 -> Mux1/1  "indicate airspeed"
  Gain2/1 -> Sqrt1/1
  Dynamic Pressure/1 -> Gain2/1
  time_usec/1 -> Bus Creator/1  "time_usec"
  Vb/1 -> dot1/1, Dynamic Pressure/1
  AngQuat/1 -> Data Type Conversion2/1
  Ve/1 -> Gain4/1
  wb/1 -> Data Type Conversion3/1
  Airspeed1/1 -> Mux1/2  "true airspeed"
  Mux1/1 -> Gain7/1
  Demux4/1 -> Bus Creator/12  "ind_airspeed"
  Demux4/2 -> Bus Creator/13  "true_airspeed"
  Demux3/3 -> Bus Creator/16  "zacc"
  Demux3/2 -> Bus Creator/15  "yacc"
  Demux3/1 -> Bus Creator/14  "xacc"
  Gain5/1 -> Data Type Conversion8/1
  Accb/1 -> Gain5/1
  Demux2/3 -> Bus Creator/11  "vz"
  Demux2/2 -> Bus Creator/10  "vy"
  Demux2/1 -> Bus Creator/9  "vx"
  Gain4/1 -> Data Type Conversion7/1
  Gain3/1 -> Data Type Conversion5/1  "alt"
  Gain1/1 -> Data Type Conversion1/1  "lon"
  Gain/1 -> Data Type Conversion4/1  "lat"
  Demux1/3 -> Gain3/1
  Demux1/2 -> Gain1/1
  Demux1/1 -> Gain/1
  Demux/3 -> Bus Creator/5  "yawspeed"
  Demux/2 -> Bus Creator/4  "pitchspeed"
  Demux/1 -> Bus Creator/3  "rollspeed"
  Data Type Conversion2/1 -> Bus Creator/2  "attitude_quaternion"
  pho/1 -> Dynamic Pressure/2
  Gain7/1 -> Data Type Conversion9/1
  dot1/1 -> Airspeed1/1
  Data Type Conversion3/1 -> Demux/1
  Data Type Conversion7/1 -> Demux2/1
  Data Type Conversion9/1 -> Demux4/1
  Data Type Conversion8/1 -> Demux3/1
  Data Type Conversion4/1 -> Bus Creator/6  "lat"
  Data Type Conversion1/1 -> Bus Creator/7  "lon"
  Data Type Conversion5/1 -> Bus Creator/8  "alt"
  Bus Creator/1 -> stateOut/1
  PosGPS/1 -> Demux1/1
